simulink model "StateflowDelivery"  (R2022a)
settings: Solver=VariableStepAuto  StartTime=0.0  StopTime=10.0  RelTol=1e-3
settings Model: Creator=31630  LastModifiedBy=31630

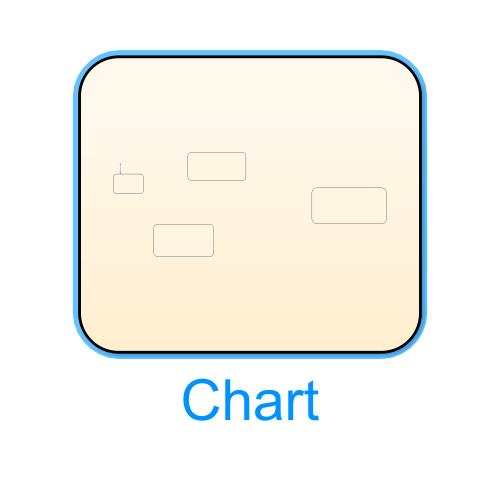
[thumbnail: Simulink's stored preview of the top-level diagram]
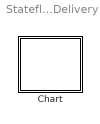
== system StateflowDelivery ==
  Chart : Stateflow chart  TreatAsAtomicUnit=on

== stateflow chart StateflowDelivery/Chart ==
  state Deliver
    entry: B = 1;
  state Takeoff
  state Land
    entry: land = 1;
  state TakePicture
    entry: objectdetected = 1;
    during: takepicture = 1;
  (default) -> Takeoff
